simulink model "ccmodels"  (R2016a)
settings: Solver=VariableStepAuto  StartTime=0.0  StopTime=120  RelTol=1e-3
undefined symbols (not defined in the file): b, m
settings Model: Creator=Admin  LastModifiedBy=Admin

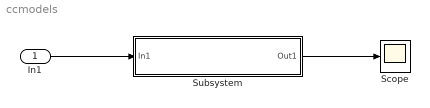
== system ccmodels ==
  In1 : Inport
  Scope : Scope
  Subsystem : Subsystem
  wires:
  In1/1 -> Subsystem/1(In1)
  Subsystem/1(Out1) -> Scope/1

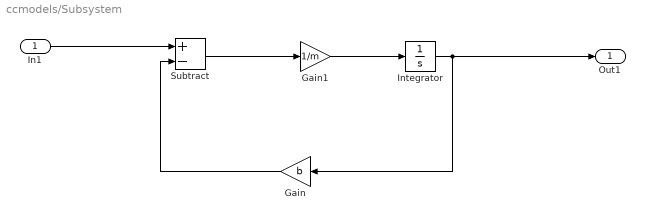
== system ccmodels/Subsystem ==
  In1 : Inport
  Gain : Gain  Gain=b
  Gain1 : Gain  Gain=1/m
  Integrator : Integrator
  Subtract : Sum  Inputs=+-
  Out1 : Outport
  wires:
  Subtract/1 -> Gain1/1
  Gain1/1 -> Integrator/1
  Integrator/1 -> Out1/1, Gain/1
  In1/1 -> Subtract/1
  Gain/1 -> Subtract/2
